simulink model "Laser_test"  (R2020a)
settings: Solver=VariableStepAuto  StartTime=0.0  StopTime=10.0  RelTol=1e-3
values from neighbouring files (symbols this model uses):
  F1 = 85005,9    [Laser.m]
  F11 = 85000    [Laser.m]
  F2 = 90000    [Laser.m]
  F3 = 94986,8    [Laser.m]
  F4 = 100000    [Laser.m]
  F5 = 115015,9    [Laser.m]
  F6 = 120000    [Laser.m]
  Te = 1/Fe    (= 3.125e-06)    [Laser.m]
settings Model: Creator=marsaa  LastModifiedBy=marsaa

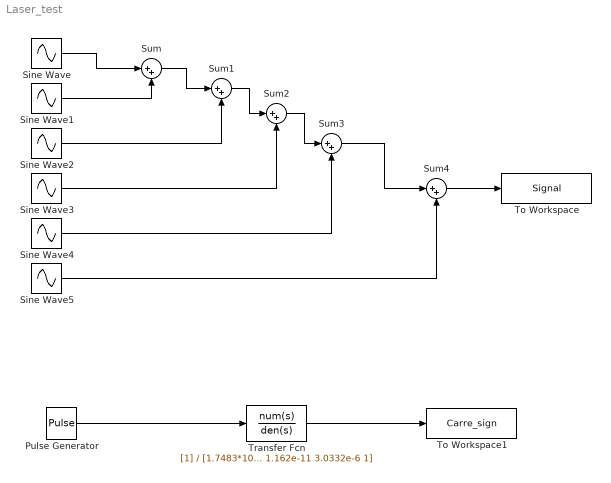
== system Laser_test ==
  Pulse Generator : DiscretePulseGenerator  PulseType=Time based  Period=1/F11  PulseWidth=50
  Sine Wave : Sin  Frequency=2*pi*F1  SampleTime=0
  Sine Wave1 : Sin  Frequency=2*pi*F2  SampleTime=0
  Sine Wave2 : Sin  Frequency=2*pi*F3  SampleTime=0
  Sine Wave3 : Sin  Frequency=2*pi*F4  SampleTime=0
  Sine Wave4 : Sin  Frequency=2*pi*F5  SampleTime=0
  Sine Wave5 : Sin  Frequency=2*pi*F6  SampleTime=0
  Sum{,1..4} (5 alike) : Sum  Inputs=|++
  To Workspace : ToWorkspace  VariableName=Signal  SaveFormat=Timeseries  SampleTime=Te
  To Workspace1 : ToWorkspace  VariableName=Carre_sign  SaveFormat=Timeseries  SampleTime=Te
  Transfer Fcn : TransferFcn  Denominator=[1.7483*10^-23 7.6663*10^-18 1.162e-11 3.0332e-6 1]
  wires:
  Sine Wave/1 -> Sum/1
  Sine Wave1/1 -> Sum/2
  Sine Wave2/1 -> Sum1/2
  Sum/1 -> Sum1/1
  Sine Wave3/1 -> Sum2/2
  Sum1/1 -> Sum2/1
  Sine Wave4/1 -> Sum3/2
  Sum2/1 -> Sum3/1
  Sine Wave5/1 -> Sum4/2
  Sum3/1 -> Sum4/1
  Sum4/1 -> To Workspace/1
  Pulse Generator/1 -> Transfer Fcn/1
  Transfer Fcn/1 -> To Workspace1/1
